simulink model "On_orbit_satellite_control_basic3"  (R2022a)
settings: Solver=ode4  StartTime=0.0  StopTime=5731  FixedStep=0.01  RelTol=1e-3
libraries: sharedtransform x5, aerolibutil x2, sharedutil x1
settings Model: Creator=sakur  LastModifiedBy=sakur

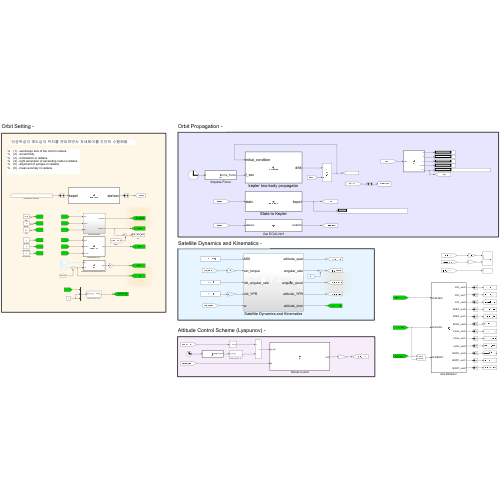
[thumbnail: Simulink's stored preview of the top-level diagram]
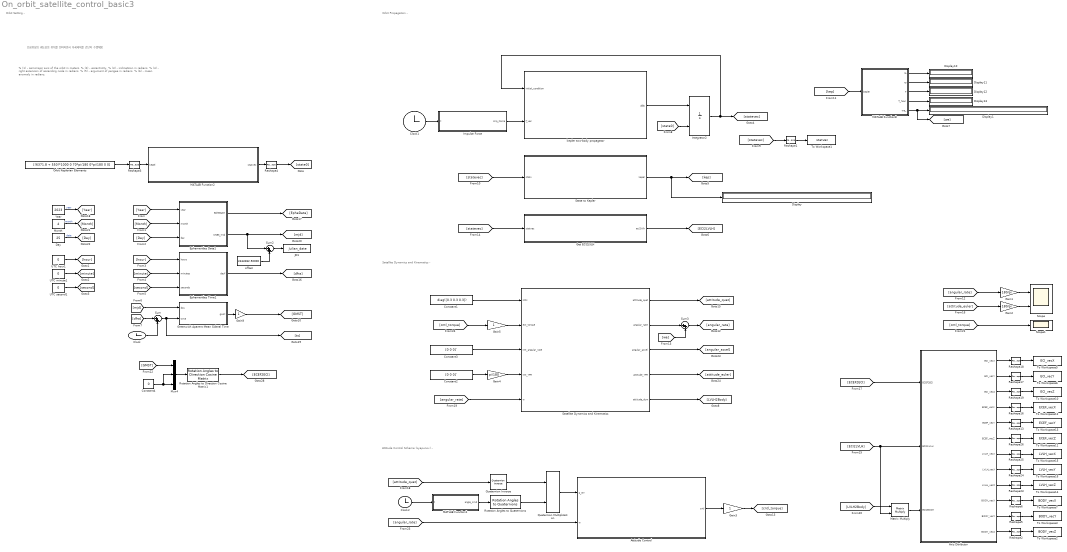
== system On_orbit_satellite_control_basic3 ==
  note: Orbit Propagation -
  note: %		(1) - semimajor axis of the orbit in meters.
      | %		(2) - eccentricity.
      | %		(3) - inclinatsion in radians.
      | %		(4) - right ascension of ascending node in radians.
      | %		(5) - argument of perigee in radians.
      | %		(6) - mean anomaly in radians.
  note: 인공위성의 궤도상의 위치를 전파하면서 자세제어를 간단히 수행해봄
  note: Attitude Control Scheme (Lyapunov) -
  note: Satellite Dynamics and Kinematics -
  note: Orbit Setting -
  Attitude Control : MATLAB Function  TreatAsAtomicUnit=on
  Axis Ditributor : MATLAB Function  TreatAsAtomicUnit=on
  Clock : Clock
  Clock1 : Clock
  Clock2 : Clock
  Constant1 : Constant  Value=diag([0.3 0.3 0.3])
  Constant2 : Constant  Value=[0 0 0]'
  Constant3 : Constant  Value=[0 0 0]'
  Constant4 : Constant  Value=0
  Day : Constant  Value=25
  Display{,1,10..13} (6 alike) : Display
  Ephemerides Date1 : Subsystem
  Ephemerides Time1 : MATLAB Function  TreatAsAtomicUnit=on
  Gain1 : Gain  Gain=180/pi
  Gain2 : Gain  Gain=180/pi
  Gain3 : Gain
  Gain4 : Gain  Gain=pi/180
  Gain5 : Gain
  Gain9 : Gain
  Get ECI2LVLH : MATLAB Function  TreatAsAtomicUnit=on
  Greenwich Aparent Mean Sideral Time : MATLAB Function  TreatAsAtomicUnit=on
  Impulse Force : MATLAB Function  TreatAsAtomicUnit=on
  Integrator2 : Integrator  InitialConditionSource=external  InitialCondition=[-7000 0 0 0 -9.175045 0 5233.5]'
  JD1 : ToWorkspace  VariableName=Julian_date  SampleTime=-1
  MATLAB Function1 : MATLAB Function  TreatAsAtomicUnit=on
  MATLAB Function2 : MATLAB Function  TreatAsAtomicUnit=on
  MATLAB Function8 : MATLAB Function  TreatAsAtomicUnit=on
  Matrix Multiply : Product  Multiplication=Matrix(*)
  Month : Constant  Value=4
  Mux4 : Mux  Inputs=3
  Orbit Keplerian Elements : Constant  Value=[(6371.8 + 550)*1000 0 70*pi/180 0*pi/180 0 0]
  Quaternion Inverse : aerolibutil/Quaternion Inverse
  Quaternion Multiplication : aerolibutil/Quaternion Multiplication
  Reshape{1..6,13,16..19,23..26} (15 alike) : Reshape  OutputDimensionality=Row vector (2-D)
  Rotation Angles to Direction Cosine Matrix1 : sharedtransform/Rotation Angles to Direction Cosine Matrix  rotationOrder=ZYX  aMode=aMode
      settings: SourceProductBaseCode=AE,PW,DR,MT,VE
  Rotation Angles to Quaternions : sharedtransform/Rotation Angles to Quaternions  rotationOrder=ZYX  aMode=aMode
      settings: SourceProductBaseCode=AE,PW,DR,MT,VE
  Satellite Dynamics and Kinematics : Subsystem
  Scope : Scope  NumInputPorts=2
  Scope1 : Scope
  State to Kepler : MATLAB Function  TreatAsAtomicUnit=on
  Sum : Sum  Inputs=|++
  Sum2 : Sum  Inputs=|++
  Sum3 : Sum  Inputs=|++
  To Workspace1 : ToWorkspace  VariableName=statvec  SampleTime=-1
      settings: Save2DSignal=2-D array (concatenate along first dimension)
  To Workspace10 : ToWorkspace  VariableName=ECI_vecZ  SampleTime=-1
      settings: Save2DSignal=2-D array (concatenate along first dimension)
  To Workspace11 : ToWorkspace  VariableName=ECEF_vecZ  SampleTime=-1
      settings: Save2DSignal=2-D array (concatenate along first dimension)
  To Workspace12 : ToWorkspace  VariableName=ECEF_vecX  SampleTime=-1
      settings: Save2DSignal=2-D array (concatenate along first dimension)
  To Workspace13 : ToWorkspace  VariableName=ECEF_vecY  SampleTime=-1
      settings: Save2DSignal=2-D array (concatenate along first dimension)
  To Workspace14 : ToWorkspace  VariableName=LVLH_vecZ  SampleTime=-1
      settings: Save2DSignal=2-D array (concatenate along first dimension)
  To Workspace15 : ToWorkspace  VariableName=LVLH_vecX  SampleTime=-1
      settings: Save2DSignal=2-D array (concatenate along first dimension)
  To Workspace16 : ToWorkspace  VariableName=LVLH_vecY  SampleTime=-1
      settings: Save2DSignal=2-D array (concatenate along first dimension)
  To Workspace2 : ToWorkspace  VariableName=BODY_vecZ  SampleTime=-1
      settings: Save2DSignal=2-D array (concatenate along first dimension)
  To Workspace3 : ToWorkspace  VariableName=BODY_vecY  SampleTime=-1
      settings: Save2DSignal=2-D array (concatenate along first dimension)
  To Workspace5 : ToWorkspace  VariableName=ECI_vecX  SampleTime=-1
      settings: Save2DSignal=2-D array (concatenate along first dimension)
  To Workspace6 : ToWorkspace  VariableName=ECI_vecY  SampleTime=-1
      settings: Save2DSignal=2-D array (concatenate along first dimension)
  To Workspace7 : ToWorkspace  VariableName=BODY_vecX  SampleTime=-1
      settings: Save2DSignal=2-D array (concatenate along first dimension)
  UTC hour1 : Constant  Value=0
  UTC minute1 : Constant  Value=0
  UTC second1 : Constant  Value=0
  Year : Constant  Value=2023
  kepler two-body propagator : MATLAB Function  TreatAsAtomicUnit=on
  offset : Constant  Value=2433282.50000
  wires:
  Reshape13/1 -> To Workspace13/1
  Constant4/1 -> Mux4/2, Mux4/3
  [GMST] -> Mux4/1
  Constant2/1 -> Gain4/1
  Constant3/1 -> Satellite Dynamics and Kinematics/3(init_angular_rate)
  Constant1/1 -> Satellite Dynamics and Kinematics/1(MOI)
  [statevec] -> Get ECI2LVLH/1(statvec)
  Axis Ditributor/2(ECI_vecY) -> Reshape17/1
  Reshape19/1 -> To Workspace10/1
  Sum2/1 -> JD1/1
  Ephemerides Date1/1(EpheDate) -> [EpheDate]
  [Month] -> Ephemerides Date1/2(month)
  Axis Ditributor/4(ECEF_vecX) -> Reshape16/1
  Reshape18/1 -> To Workspace5/1
  Axis Ditributor/9(LVLH_vecZ) -> Reshape23/1
  Clock1/1 -> Impulse Force/1(t)
  Year/1 -> [Year]  "year"
  Reshape3/1 -> MATLAB Function2/1(kepel)
  [state0] -> Integrator2/2
  Axis Ditributor/1(ECI_vecX) -> Reshape18/1
  UTC second1/1 -> [second]
  Axis Ditributor/8(LVLH_vecY) -> Reshape24/1
  Reshape17/1 -> To Workspace6/1
  Axis Ditributor/6(ECEF_vecZ) -> Reshape26/1
  [minute] -> Ephemerides Time1/2(minutes)
  Axis Ditributor/5(ECEF_vecY) -> Reshape13/1
  MATLAB Function8/2(rp) -> Display11/1
  Reshape25/1 -> To Workspace15/1
  [statevec] -> Reshape1/1
  Reshape24/1 -> To Workspace16/1
  MATLAB Function2/1(statvec) -> Reshape4/1
  [kep] -> MATLAB Function8/1(kepler)
  Reshape1/1 -> To Workspace1/1
  MATLAB Function8/5(we_) -> [we], Display1/1
  MATLAB Function8/1(ra) -> Display10/1
  Integrator2/1 -> [statevec], kepler two-body propagator/1(initial_condition)
  State to Kepler/1(kepel) -> Display/1, [kep]
  UTC hour1/1 -> [hour]
  [mjd] -> Greenwich Aparent Mean Sideral Time/1(diju)
  Get ECI2LVLH/1(eci2lvlh) -> [ECI2LVLH]
  Sum/1 -> Greenwich Aparent Mean Sideral Time/2(time), [ts]
  kepler two-body propagator/1(dfdt) -> Integrator2/1
  MATLAB Function8/4(T_hour) -> Display13/1
  Ephemerides Time1/1(dayf) -> [dfra]
  Orbit Keplerian Elements/1 -> Reshape3/1
  Gain9/1 -> [GMST]
  Rotation Angles to Direction Cosine Matrix1/1 -> [ECEF2ECI]
  [dfra] -> Sum/1
  Clock/1 -> Sum/2
  Ephemerides Date1/2(CNES_mdj) -> Sum2/1, [mjd]
  Reshape4/1 -> [state0]
  Greenwich Aparent Mean Sideral Time/1(gwst) -> Gain9/1
  Impulse Force/1(Imp_Force) -> kepler two-body propagator/2(f_vec)
  Axis Ditributor/3(ECI_vecZ) -> Reshape19/1
  [Day] -> Ephemerides Date1/3(day)
  Month/1 -> [Month]  "month"
  [ECEF2ECI] -> Axis Ditributor/1(ECEF2ECI)
  Day/1 -> [Day]  "date"
  offset/1 -> Sum2/2
  MATLAB Function8/3(T) -> Display12/1
  Reshape26/1 -> To Workspace11/1
  [hour] -> Ephemerides Time1/1(hours)
  Reshape16/1 -> To Workspace12/1
  [second] -> Ephemerides Time1/3(seconds)
  Mux4/1 -> Rotation Angles to Direction Cosine Matrix1/1
  UTC minute1/1 -> [minute]
  Axis Ditributor/7(LVLH_vecX) -> Reshape25/1
  [Year] -> Ephemerides Date1/1(year)
  [statevec] -> State to Kepler/1(statv)
  Reshape23/1 -> To Workspace14/1
  Reshape2/1 -> To Workspace2/1
  Axis Ditributor/12(BODY_vecZ) -> Reshape2/1
  Reshape5/1 -> To Workspace3/1
  Axis Ditributor/11(BODY_vecY) -> Reshape5/1
  Reshape6/1 -> To Workspace7/1
  Axis Ditributor/10(BODY_vecX) -> Reshape6/1
  [ECI2LVLH] -> Matrix Multiply/2, Axis Ditributor/2(ECI2LVLH)
  Matrix Multiply/1 -> Axis Ditributor/3(ECI2BODY)
  [LVLH2Body] -> Matrix Multiply/1
  [angular_rate] -> Satellite Dynamics and Kinematics/5(w)
  [angular_rate] -> Gain1/1
  [attitude_euler] -> Gain2/1
  Gain2/1 -> Scope/2
  Gain1/1 -> Scope/1
  Gain4/1 -> Satellite Dynamics and Kinematics/4(Init_YPR)
  Sum3/1 -> [angular_rate]
  [we] -> Sum3/2
  Satellite Dynamics and Kinematics/2(angular_rate) -> Sum3/1
  Satellite Dynamics and Kinematics/5(attitude_dcm) -> [LVLH2Body]
  Satellite Dynamics and Kinematics/1(attitude_quat) -> [attitude_quat]
  Satellite Dynamics and Kinematics/3(angular_accel) -> [angular_accel]
  Satellite Dynamics and Kinematics/4(attitude_YPR) -> [attitude_euler]
  [angular_rate] -> Attitude Control/2(w)
  Attitude Control/1(cntl) -> Gain3/1
  [cntl_torque] -> Gain5/1
  Quaternion Multiplication/1 -> Attitude Control/1(q_err)
  [attitude_quat] -> Quaternion Inverse/1
  Quaternion Inverse/1 -> Quaternion Multiplication/1
  Rotation Angles to Quaternions/1 -> Quaternion Multiplication/2
  Gain3/1 -> [cntl_torque]
  Clock2/1 -> MATLAB Function1/1(t)
  MATLAB Function1/1(angle_cmd) -> Rotation Angles to Quaternions/1
  Gain5/1 -> Satellite Dynamics and Kinematics/2(ext_torque)
  [cntl_torque] -> Scope1/1

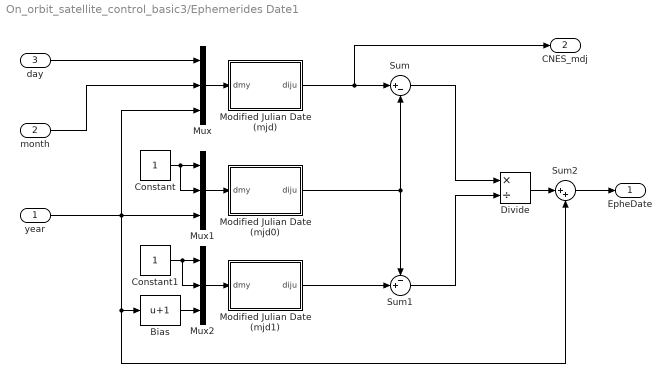
== system On_orbit_satellite_control_basic3/Ephemerides Date1 ==
  year : Inport
  month : Inport  Port=2
  day : Inport  Port=3
  Bias : Bias  Bias=1  SaturateOnIntegerOverflow=off
  Constant : Constant
  Constant1 : Constant
  Divide : Product  Inputs=*/
  Modified Julian Date (mjd) : MATLAB Function  TreatAsAtomicUnit=on
  Modified Julian Date (mjd0) : MATLAB Function  TreatAsAtomicUnit=on
  Modified Julian Date (mjd1) : MATLAB Function  TreatAsAtomicUnit=on
  Mux : Mux  Inputs=3
  Mux1 : Mux  Inputs=3
  Mux2 : Mux  Inputs=3
  Sum : Sum  Inputs=|+-
  Sum1 : Sum  Inputs=-+|
  Sum2 : Sum  Inputs=|++
  EpheDate : Outport
  CNES_mdj : Outport  Port=2
  wires:
  Sum1/1 -> Divide/2
  Modified Julian Date (mjd1)/1(diju) -> Sum1/2
  month/1 -> Mux/2
  year/1 -> Mux1/3, Mux/3, Bias/1, Sum2/2
  Mux1/1 -> Modified Julian Date (mjd0)/1(dmy)
  day/1 -> Mux/1
  Mux/1 -> Modified Julian Date (mjd)/1(dmy)
  Mux2/1 -> Modified Julian Date (mjd1)/1(dmy)
  Bias/1 -> Mux2/3
  Modified Julian Date (mjd)/1(diju) -> CNES_mdj/1, Sum/1
  Constant1/1 -> Mux2/2, Mux2/1
  Sum/1 -> Divide/1
  Constant/1 -> Mux1/2, Mux1/1
  Modified Julian Date (mjd0)/1(diju) -> Sum1/1, Sum/2
  Divide/1 -> Sum2/1
  Sum2/1 -> EpheDate/1

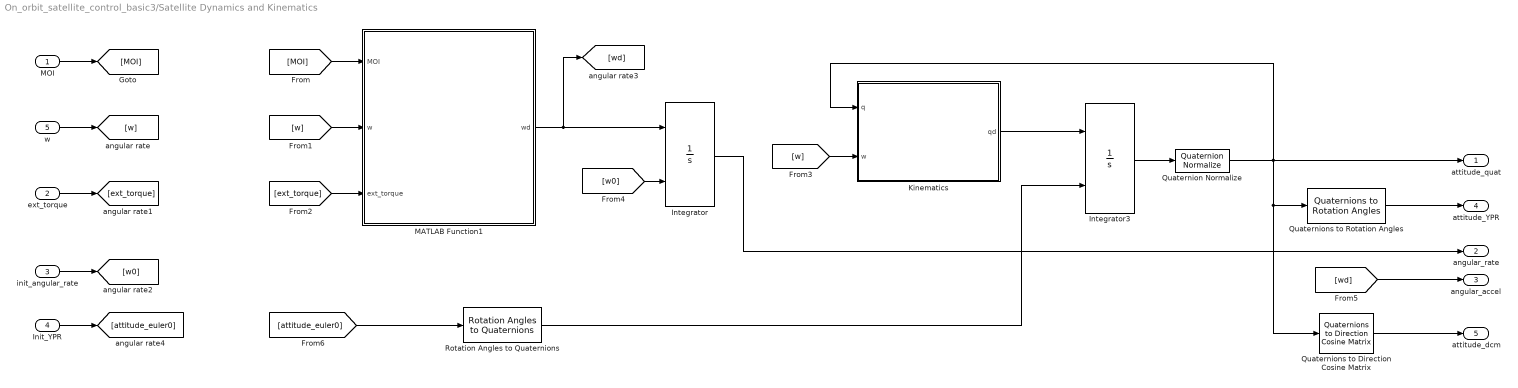
== system On_orbit_satellite_control_basic3/Satellite Dynamics and Kinematics ==
  MOI : Inport
  ext_torque : Inport  Port=2
  init_angular_rate : Inport  Port=3
  Init_YPR : Inport  Port=4
  w : Inport  Port=5
  Integrator : Integrator  InitialConditionSource=external
  Integrator3 : Integrator  InitialConditionSource=external
  Kinematics : MATLAB Function  TreatAsAtomicUnit=on
  MATLAB Function1 : MATLAB Function  TreatAsAtomicUnit=on
  Quaternion Normalize : sharedutil/Quaternion Normalize  aMode=aMode
      settings: SourceProductBaseCode=AE,PW,DR,MT,VE
  Quaternions to Direction Cosine Matrix : sharedtransform/Quaternions to  Direction Cosine Matrix  aMode=aMode
      settings: SourceProductBaseCode=AE,PW,DR,MT,VE
  Quaternions to Rotation Angles : sharedtransform/Quaternions to Rotation Angles  rotationOrder=ZYX  aMode=aMode
      settings: SourceProductBaseCode=AE,PW,DR,MT,VE
  Rotation Angles to Quaternions : sharedtransform/Rotation Angles to Quaternions  rotationOrder=ZYX  aMode=aMode
      settings: SourceProductBaseCode=AE,PW,DR,MT,VE
  attitude_quat : Outport
  angular_rate : Outport  Port=2
  angular_accel : Outport  Port=3
  attitude_YPR : Outport  Port=4
  attitude_dcm : Outport  Port=5
  wires:
  Kinematics/1(qd) -> Integrator3/1
  Quaternion Normalize/1 -> Kinematics/1(q), attitude_quat/1, Quaternions to Direction Cosine Matrix/1, Quaternions to Rotation Angles/1
  Rotation Angles to Quaternions/1 -> Integrator3/2
  Integrator3/1 -> Quaternion Normalize/1
  MATLAB Function1/1(wd) -> [wd], Integrator/1
  Quaternions to Rotation Angles/1 -> attitude_YPR/1
  Quaternions to Direction Cosine Matrix/1 -> attitude_dcm/1
  Integrator/1 -> angular_rate/1
  MOI/1 -> [MOI]
  [MOI] -> MATLAB Function1/1(MOI)
  w/1 -> [w]
  ext_torque/1 -> [ext_torque]
  [w] -> MATLAB Function1/2(w)
  [ext_torque] -> MATLAB Function1/3(ext_torque)
  [w] -> Kinematics/2(w)
  init_angular_rate/1 -> [w0]
  [w0] -> Integrator/2
  [wd] -> angular_accel/1
  Init_YPR/1 -> [attitude_euler0]
  [attitude_euler0] -> Rotation Angles to Quaternions/1

== matlab function On_orbit_satellite_control_basic3/Ephemerides Date1/Modified Julian Date (mjd0) ==
  data: dmy input; diju output
function diju  =  djm (dmy)
% [diju] = djm (day, month, year)
%    The function djm furnishes the Modified Julian
%    Date with reference to the day, month and year,
%    at zero hours of the day.
% inputs:
%   dmy(1): day, day of the month
%   dmy(2): month, month of the year
%   dmy(3): year

% outputs:
%   diju
%       Modified Julian Date in days, referred to 1950.0. 
%
% Valdemir Carrara, Apr, 2003
%

diju = 367*dmy(3) + dmy(1) - 712269 + fix(275*dmy(2)/9)- fix(7*(dmy(3)+fix((dmy(2)+9)/12))/4);

== matlab function On_orbit_satellite_control_basic3/Ephemerides Date1/Modified Julian Date (mjd1) ==
  data: dmy input; diju output
function diju  =  djm (dmy)
% [diju] = djm (day, month, year)
%    The function djm furnishes the Modified Julian
%    Date with reference to the day, month and year,
%    at zero hours of the day.
% inputs:
%   dmy(1): day, day of the month
%   dmy(2): month, month of the year
%   dmy(3): year

% outputs:
%   diju
%       Modified Julian Date in days, referred to 1950.0. 
%
% Valdemir Carrara, Apr, 2003
%

diju = 367*dmy(3) + dmy(1) - 712269 + fix(275*dmy(2)/9)- fix(7*(dmy(3)+fix((dmy(2)+9)/12))/4);

== matlab function On_orbit_satellite_control_basic3/Ephemerides Time1 ==
  data: hours input; dayf output; minutes input; seconds input
function dayf  = time_to_dayf(hours, minutes, seconds)
% [dayf] = time_to_dayf (hours, minutes, seconds)
%    The function time_to_dayf returns with the day elapesed
%    time in seconds
% inputs:
%   hours     
%       day hour (integer).
%   minutes
%       minutes (integer).
%   seconds
%       seconds and fraction of second
% outputs:
%   dayf
%       Day elapsed time in seconds. 
%
% Valdemir Carrara, Feb, 2009
%

dayf = seconds + 60*(minutes + 60*hours);

== matlab function On_orbit_satellite_control_basic3/MATLAB Function8 ==
  data: kepler input; ra output; rp output; T output; T_hour output; we_ output
function [ra, rp, T, T_hour, we_] = fcn(kepler)

u=3.9865*10^14;

a = kepler(1);
e = kepler(2);
% 

ra = a*(1+e);%장반경
rp = a*(1-e);%단반경

a = (ra+rp)/2;% semi-major axis

% a = (550 + 6371.8)*1000;

T = 2*pi*sqrt((a*a*a)/(u));% 1 궤도 주기

T_hour = T/3600;

we = 2*pi/T;

we_ = [0 we 0]';%LVLH frame에서 y축이 궤도와 수직함, 즉 y축이 곧 회전축이라 이러헥 정의

end

== matlab function On_orbit_satellite_control_basic3/Satellite Dynamics and Kinematics/Kinematics ==
  data: q input; qd output; w input
function qd    = kinematics( q, w )
w1 = w(1);  w2 = w(2);  w3 = w(3);

Omega = [ 0 -w1 -w2 -w3; 
         w1   0  w3 -w2;
         w2 -w3   0  w1;
         w3  w2 -w1   0];

qd = 0.5*Omega*q;


end

== matlab function On_orbit_satellite_control_basic3/Get ECI2LVLH ==
  data: statvec input; eci2lvlh output
function eci2lvlh  = fcn(statvec)
r = statvec(1:3)';% wrt eci
v = statvec(4:6)';% wrt eci

LVLH_Z = -r/norm(r);
LVLH_Y = -cross(v,LVLH_Z)/norm(cross(v,LVLH_Z));
LVLH_X =  cross(LVLH_Y, LVLH_Z);

eci2lvlh = [LVLH_X,LVLH_Y,LVLH_Z]';

end

== matlab function On_orbit_satellite_control_basic3/Satellite Dynamics and Kinematics/MATLAB Function1 ==
  data: MOI input; wd output; w input; ext_torque input
function wd = Dynamics(MOI, w, ext_torque)

wd = inv(MOI)*(ext_torque - cross(w, MOI*w));

end

== matlab function On_orbit_satellite_control_basic3/kepler two-body propagator ==
  data: initial_condition input; dfdt output; f_vec input
function dfdt  = eq_propagate(initial_condition, f_vec)

u  = 3.9865*10^14;
Re = 6378137; % earth radius in m
sat_mass = 100;%[kg]

dfdt = zeros(size(initial_condition));

x1 = initial_condition(4); % x1 = dx/dt
y1 = initial_condition(5); % y1 = dy/dt
z1 = initial_condition(6); % z1 = dz/dt
x  = initial_condition(1); % x
y  = initial_condition(2); % y
z  = initial_condition(3); % z

r=sqrt(x^2+y^2+z^2);

% % %   Keplar Motion Equatnion
% % %  => r_dd + u/(r^3)r_ = 0 => r_dd = -u/(r^3)r_
dfdt(1) = x1;
dfdt(2) = y1;
dfdt(3) = z1;
dfdt(4) = -u*x/r^3 + f_vec(1)/sat_mass;
dfdt(5) = -u*y/r^3 + f_vec(2)/sat_mass;
dfdt(6) = -u*z/r^3 + f_vec(3)/sat_mass;

end

== matlab function On_orbit_satellite_control_basic3/MATLAB Function2 ==
  data: kepel input; statvec output
function statvec  = kepel_statvec (kepel)
%  [statvec] = kepel_statvec (kepel)
%	The function kepel_statvec transforms the keplerian
%	elements kepel into the corresponding state vector in
%	the same reference system.
%
% Input:
%	kepel
% 		vector containing the keplerian elements:
%		(1) - semimajor axis of the orbit in meters.
%		(2) - eccentricity.
%		(3) - inclinatsion in radians.
%		(4) - right ascension of ascending node in radians.
%		(5) - argument of perigee in radians.
%		(6) - mean anomaly in radians.
% Output:
%	statvec
%  		state vector in meters and meters/second.
%
% Authors:
%	Helio K. Kuga;
%	Valder M. Medeiros;
%	Valdemir Carrara		february/80		version 1.0
%	Valdemir Carrara		july 2005		(C version)
%   Valdemir Carrara            March/09        Matlab

EARTH_GRAVITY	= 3.9860064e+14;		% Earth's gravitational constant (m**3/s**2)

a    = kepel(1);	% semi-major axis
exc  = kepel(2);	% eccentricity

c1   = sqrt(1. - exc*exc);

%     rotation matrix

orb2iner = rotmaz(-kepel(4))*rotmax(-kepel(3))*rotmaz(-kepel(5));

%     Kepler's equation

E    = kepler(kepel(6), exc);

sE   = sin(E);
cE   = cos(E);
c3   = sqrt(EARTH_GRAVITY/a)/(1. - exc*cE);

%     state vector

statvec = [[a*(cE - exc), a*c1*sE, 0]*orb2iner', [-c3*sE, c1*c3*cE, 0]*orb2iner'];

end

function [rot_mat] = rotmax (angle)
% [rot_mat] = rotmax (angle)
%   To obtain the rotation matrix around the X axis given the
%   rotation angle.
% inputs:
%   angle
%       rotation angle, in radians.
% outputs:
%   rot_mat
%       rotation matrix (3, 3)
%

% Valdemir Carrara, Sep, 1998

coan    =  cos(angle);
sian    =  sin(angle);

rot_mat =  [1, 0, 0; 0, coan, sian; 0, -sian, coan];

end

function [rot_mat] = rotmay (angle)
% [rot_mat] = rotmay (angle)
%   To obtain the rotation matrix around the Y axis given the
%   rotation angle.
% inputs:
%   angle
%       rotation angle, in radians.
% outputs:
%   rot_mat
%       rotation matrix (3, 3)
%

% Valdemir Carrara, Sep, 1998


coan    =  cos(angle);
sian    =  sin(angle);

rot_mat =  [coan, 0, -sian; 0, 1, 0; sian, 0, coan];

end

function [rot_mat] = rotmaz (angle)
% [rot_mat] = rotmaz (angle)
%   To obtain the rotation matrix around the Z axis given the
%   rotation angle.
% inputs:
%   angle
%       rotation angle, in radians.
% outputs:
%   rot_mat
%       rotation matrix (3, 3)
%

% Valdemir Carrara, Sep, 1998

coan    =  cos(angle);
sian    =  sin(angle);

rot_mat =  [coan, sian, 0; -sian, coan, 0; 0, 0, 1];
end

function [eccentric] = kepler (mean_anomaly, eccentricity)
% [eccentric] = kepler (mean_anomaly, eccentricity)
%	The subroutine kepler finds a solution to the
%	kepler's equation.
%
% Input:
%	mean_anomaly
%		mean anomaly in radians.
%	eccentricity
%		eccentricity.
%
% Output:
%	eccentric
%		eccentric anomaly in radians.
%
% Authors:
%	Valder M. de Medeiros		june/81		version 2.0
%	Valdemir Carrara			july 2005	(C version)
%   Valdemir Carrara            March/09        Matlab

exc2    = eccentricity*eccentricity;
am1     = mod (mean_anomaly, 2*pi);
am2     = am1 + am1;
am3     = am1 + am2;
shoot   = am1 + eccentricity*(1. - 0.125*exc2)*sin(am1) + ...
		0.5*exc2*(sin(am2) + 0.75*eccentricity*sin(am3));
shoot   = mod (shoot, 2*pi);

e1      = 1.0;
ic      = 0;

while ((abs(e1) > 1.e-12) && (ic <= 10)) 
	e1    = (shoot - am1 - eccentricity*sin(shoot)) / ...
			(1.0 - eccentricity*cos(shoot));
    shoot = shoot - e1;
    ic    = ic + 1;
end

if (ic >= 10)
    disp ('warning ** subroutine kepler did not converge in 10 iterations');
end

eccentric = shoot;


end

== matlab function On_orbit_satellite_control_basic3/Attitude Control ==
  data: q_err input; cntl output; w input
function cntl = fcn(q_err, w)


qe_w = q_err(  1,1);
qe_v = q_err(2:4,1);

K1 = diag([0.1 0.1 0.1]);
K2 = diag([0.3 0.3 0.3]);

cntl = K1*qe_v - K2*w;

end

== matlab function On_orbit_satellite_control_basic3/Impulse Force ==
  settings: updateMethod=DISCRETE
  data: Imp_Force output; t input
function Imp_Force  = fcn(t)

Imp_Force = [0 0 0]';

% if ((t >= 1000) && (t <= 1050))
%     Imp_Force =  [10000 0 20000]';
% elseif ((t >= 1100) && (t <= 1150))
%     Imp_Force = -[-20000 0 10000]';
% else
%     Imp_Force = [0 0 0]';
% 
% end

end

== matlab function On_orbit_satellite_control_basic3/State to Kepler ==
  settings: updateMethod=DISCRETE
  data: statv input; kepel output
function kepel  = statvec_kepel (statv)
%	The function statvec_kepel transforms the state vector statv
%	into the corresponding keplerian elements in the
%	same reference system.
%
% Input:
%	statv
%		state vector in meters and meters/second.
%
% Output:
%	statvec_kepel
%		vector containing the keplerian elements:
%		(1) - semimajor axis of the orbit in meters.
%		(2) - eccentricity.
%		(3) - inclination in radians.
%		(4) - right ascension of ascending node in radians.
%		(5) - argument of perigee in radians.
%		(6) - mean anomaly in radians.

EARTH_GRAVITY	= 3.9860064e+14;		% Earth's gravitational constant (m**3/s**2)

xp     = [statv(1),statv(2),statv(3)];
xv     = [statv(4),statv(5),statv(6)];
r      = sqrt(xp*xp');
vq     = xv*xv';
ainv   = 2.0/(r) - vq/EARTH_GRAVITY;

if ainv <= 0
%     pause(1);
    ainv=0;
end

h      = cross(xp, xv);
hm     = sqrt(h*h');

if (hm < 1.e-10)
    disp (' *** Message from function statvec_kepel: *** ');
    disp (' There are no keplerian elements corresponding to this state vector');
    kepel = [0, 0, 0, 0, 0, 0];
else
    h      = h/hm;
    incl   = acos(h(3));
    raan   = atan2(h(1), -h(2));
    d      = xp*xv' / EARTH_GRAVITY;
    esene  = d * sqrt(EARTH_GRAVITY*ainv);
    ecose  = 1 - r*ainv;
    exc    = sqrt(esene*esene + ecose*ecose);
    E      = atan2(esene, ecose);
    mean   = mod (E - esene, 2*pi);
    an = [0 0 0];
    if mean < 0
        mean = mean + 2*pi;
    end
    if exc < 1.e-10
        arpe = 0;
    else
        dp     = 1./r - ainv;
        ev     = dp*xp - d*xv;
        abev   = sqrt(ev*ev');
        ev     = ev/abev;
        an(1)  = cos(raan);
        an(2)  = sin(raan);
        an(3)  = 0;
        fi     = ev*cross(h, an)';
        arpe = acos(ev*an');
        if fi < 0
            arpe  =  -arpe + 2*pi;
        end
    end

    kepel = [(1./ainv), exc, incl, raan, arpe, mean];
    kepel_save = kepel;
    %         T = 2*pi*sqrt((a*a*a)/(EARTH_GRAVITY));
end


end

== matlab function On_orbit_satellite_control_basic3/MATLAB Function1 ==
  data: t input; angle_cmd output
function angle_cmd = fcn(t)

angle_cmd = [0 0 10*sin(0.01*t)]'*pi/180;%[yaw pitch roll]

end

== matlab function On_orbit_satellite_control_basic3/Greenwich Aparent Mean Sideral Time ==
  data: diju input; gwst output; time input
function gwst  = gst (diju, time)
% [gwst] = gst (diju, time)
%   The function gst furnishes the greenwich aparent mean 
%   sidereal time referred to the J2000.0 equator and equinox.
% inputs:
%   diju
%       Modified Julian Date in days, referred to 1950.0.
%   time
%       UT1 time complement in seconds.
% outputs:
%   gwst
%       Greenwich aparent sidereal time in radians
%
% Valdemir Carrara, Apr, 2003
%

tsj = (diju-18262.5)/36525;
tsgo = (24110.54841 + (8640184.812866 + 9.3104e-2*tsj - 6.2e-6*tsj*tsj)*tsj)*pi/43200;
tetp = 7.292116e-5;		% velocidade angular da Terra (rd/s) mean angular velocity of the Earth
gwst = mod(tsgo + time*tetp, 2*pi);
% reference site
% https://www2.mps.mpg.de/homes/fraenz/systems/systems2art/node10.html
%      if (gwst<0) gwst = gwst + 2*pi

== matlab function On_orbit_satellite_control_basic3/Ephemerides Date1/Modified Julian Date (mjd) ==
  data: dmy input; diju output
function diju  =  djm (dmy)
% [diju] = djm (day, month, year)
%    The function djm furnishes the Modified Julian
%    Date with reference to the day, month and year,
%    at zero hours of the day.
% inputs:
%   dmy(1): day, day of the month
%   dmy(2): month, month of the year
%   dmy(3): year

% outputs:
%   diju
%       Modified Julian Date in days, referred to 1950.0. 
%
% Valdemir Carrara, Apr, 2003
%

diju = 367*dmy(3) + dmy(1) - 712269 + fix(275*dmy(2)/9)- fix(7*(dmy(3)+fix((dmy(2)+9)/12))/4);

== matlab function On_orbit_satellite_control_basic3/Axis Ditributor ==
  data: ECEF2ECI input; ECI_vecX output; ECI_vecY output; ECI_vecZ output; ECEF_vecX output; ECEF_vecY output; ECEF_vecZ output; LVLH_vecX output; LVLH_vecY output; LVLH_vecZ output; ECI2LVLH input; ECI2BODY input; BODY_vecX output; BODY_vecY output; BODY_vecZ output
function [ ECI_vecX,  ECI_vecY,  ECI_vecZ,...
          ECEF_vecX, ECEF_vecY, ECEF_vecZ,...
          LVLH_vecX, LVLH_vecY, LVLH_vecZ,...
          BODY_vecX, BODY_vecY, BODY_vecZ] = ...
          fcn(ECEF2ECI, ECI2LVLH, ECI2BODY)

ECI_vecX  = [5000000, 0, 0]';
ECI_vecY  = [0, 5000000, 0]';
ECI_vecZ  = [0, 0, 5000000]';

ECEF_vecX = ECEF2ECI'*ECI_vecX;
ECEF_vecY = ECEF2ECI'*ECI_vecY;
ECEF_vecZ = ECEF2ECI'*ECI_vecZ;

sc=0.5;
LVLH_vecX = ECI2LVLH'*ECI_vecX*sc;
LVLH_vecY = ECI2LVLH'*ECI_vecY*sc;
LVLH_vecZ = ECI2LVLH'*ECI_vecZ*sc;

BODY_vecX = ECI2BODY'*ECI_vecX*sc;
BODY_vecY = ECI2BODY'*ECI_vecY*sc;
BODY_vecZ = ECI2BODY'*ECI_vecZ*sc;
% BODY_vecX = LVLH2BODY(:,1)*500000;
% BODY_vecY = LVLH2BODY(:,2)*500000;
% BODY_vecZ = LVLH2BODY(:,3)*500000;


end
